simulink model "Proiect_3_sim"  (R2025b)
settings: Solver=VariableStepAuto  StartTime=0.0  StopTime=10.0  RelTol=1e-3
libraries: slpidlib x1
settings Model: Creator=Rares  LastModifiedBy=Rares

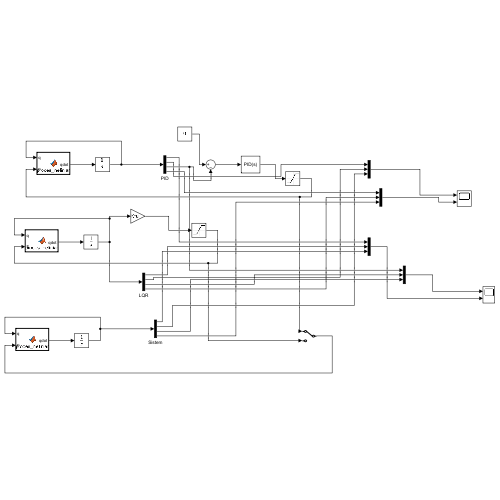
[thumbnail: Simulink's stored preview of the top-level diagram]
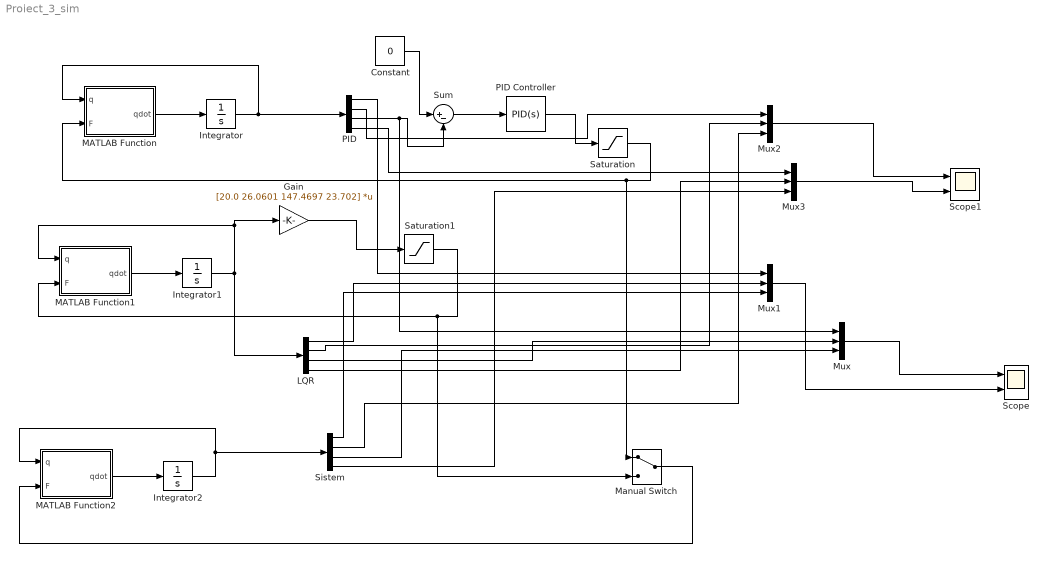
== system Proiect_3_sim ==
  Constant : Constant  Value=0
  Gain : Gain  Gain=[20.0 26.0601 147.4697 23.702]  Multiplication=Matrix(K*u)
  Integrator : Integrator  InitialCondition=[0;0;0.5;0]
  Integrator1 : Integrator  InitialCondition=[0;0;0.5;0]
  Integrator2 : Integrator  InitialCondition=[0;0;0.5;0]
  LQR : Demux
  MATLAB Function : MATLAB Function  TreatAsAtomicUnit=on
  MATLAB Function1 : MATLAB Function  TreatAsAtomicUnit=on
  MATLAB Function2 : MATLAB Function  TreatAsAtomicUnit=on
  Manual Switch : ManualSwitch
  Mux{,1..3} (4 alike) : Mux  Inputs=3
  PID : Demux
  PID Controller : slpidlib/PID Controller  Controller=PID  Form=Parallel  TimeDomain=Continuous-time  UseExternalTs=off  SampleTime=-1  IntegratorMethod=Forward Euler  FilterMethod=Forward Euler  ControllerParametersSource=internal  P=-12.8009  I=-6.9217  UseKiTs=off  D=-1.9402  UseExternalDerivativeSource=off  N=100  UseFilter=on  TunerSelectOption=Transfer Function Based (PID Tuner App)  InitialConditionSource=internal  InitialConditionForIntegrator=0  InitialConditionForFilter=0  DifferentiatorICPrevScaledInput=0  ExternalReset=none  TrackingMode=off  Kt=1  LimitOutput=off  SatLimitsSource=internal  UpperSaturationLimit=inf  LowerSaturationLimit=-inf  LinearizeAsGain=on  AntiWindupMode=none  Kb=1  LimitIntegrator=off  UpperIntegratorSaturationLimit=inf  LowerIntegratorSaturationLimit=-inf  POutMin=[]  POutMax=[]  IOutMin=[]  IOutMax=[]  DOutMin=[]  DOutMax=[]  NOutMin=[]  NOutMax=[]  SumOutMin=[]  SumOutMax=[]  SaturationOutMin=[]  SaturationOutMax=[]  PParamMin=[]  PParamMax=[]  IParamMin=[]  IParamMax=[]  DParamMin=[]  DParamMax=[]  NParamMin=[]  NParamMax=[]  KbParamMin=[]  KbParamMax=[]  KtParamMin=[]  KtParamMax=[]  KbOutMin=[]  KbOutMax=[]  KtOutMin=[]  KtOutMax=[]  IntegratorOutMin=[]  IntegratorOutMax=[]  FilterOutMin=[]  FilterOutMax=[]  SumI1OutMin=[]  SumI1OutMax=[]  SumI2OutMin=[]  SumI2OutMax=[]  SumI3OutMin=[]  SumI3OutMax=[]  SumI4OutMin=[]  SumI4OutMax=[]  SumDOutMin=[]  SumDOutMax=[]  DifferentiatorOutMin=[]  DifferentiatorOutMax=[]  FilterDiffOutCoefMin=[]  FilterDiffOutCoefMax=[]  ReciprocalOutMin=[]  ReciprocalOutMax=[]  SumDenOutMin=[]  SumDenOutMax=[]  SumNumOutMin=[]  SumNumOutMax=[]  DivideOutMin=[]  DivideOutMax=[]  UdiffTsProdOutMin=[]  UdiffTsProdOutMax=[]  NTsProdOutMin=[]  NTsProdOutMax=[]  UintegralTsProdOutMin=[]  UintegralTsProdOutMax=[]  UngainTsProdOutMin=[]  UngainTsProdOutMax=[]  ClampingZeroOutDataTypeStr=Inherit: Inherit via back propagation  ClampingZeroOutMin=[]  ClampingZeroOutMax=[]  FilterDenConstantOutDataTypeStr=Inherit: Inherit via back propagation  FilterDenConstantOutMin=[]  FilterDenConstantOutMax=[]  PCopyOutDataTypeStr=Inherit: Inherit via back propagation  PCopyOutMin=[]  PCopyOutMax=[]  NCopyOutDataTypeStr=Inherit: Inherit via back propagation  NCopyOutMin=[]  NCopyOutMax=[]  IntegratorContinuousStateAttributes=''  IntegratorStateMustResolveToSignalObject=off  IntegratorRTWStateStorageClass=Auto  FilterContinuousStateAttributes=''  FilterStateMustResolveToSignalObject=off  FilterRTWStateStorageClass=Auto  ParallelPVariant=InternalParameters  IdealPVariant=Disabled  IVariant=InternalParameters  DVariant=InternalParameters  IntegratorVariant=Continuous  SatVariant=Disabled  AWVariant=Passthrough  PCopyVariant=Disabled  TRVariant=Disabled  FdbkBlocksVariant=Forward  IdealPFdbkVariant=Disabled  SatFdbkVariant=Disabled  DerivativeFilterVariant=ContFilter  NVariant=InternalParameters  NCopyVariant=Disabled  FilterICVariant=InternalICsFilter  IntegratorICVariant=InternalICs  ExternalResetVariant=Disabled  TRSumVariant=Passthrough  SumFdbkVariant=Disabled  SumVariant=Sum_PID  TsampFilterVariant=InternalTs  TsampNgainVariant=Passthrough  TsampIntegralVariant=Disabled_SignalSpec  ExternalSaturationOutDataTypeStr=Inherit: Same as second input  DerivativeSourceVariant=ErrorSignal  PreIntVariant=InternalPreInt
  Saturation : Saturate  UpperLimit=10  LowerLimit=-10
  Saturation1 : Saturate  UpperLimit=10  LowerLimit=-10
  Scope : Scope  NumInputPorts=2
      settings: ActiveDisplayYMinimum=-0.23429520453930819  ActiveDisplayYMaximum=0.5815883560599231
  Scope1 : Scope  NumInputPorts=2
      settings: ActiveDisplayYMinimum=-4.4566103795185814  ActiveDisplayYMaximum=2.4235967168961703
  Sistem : Demux
  Sum : Sum  Inputs=|+-
  wires:
  MATLAB Function/1(qdot) -> Integrator/1
  Integrator/1 -> PID/1, MATLAB Function/1(q)
  Constant/1 -> Sum/1
  PID/3 -> Mux/1, Sum/2
  PID Controller/1 -> Saturation/1
  Saturation/1 -> Manual Switch/1, MATLAB Function/2(F)
  Sum/1 -> PID Controller/1
  Integrator1/1 -> Gain/1, MATLAB Function1/1(q), LQR/1
  MATLAB Function1/1(qdot) -> Integrator1/1
  Gain/1 -> Saturation1/1
  Saturation1/1 -> Manual Switch/2, MATLAB Function1/2(F)
  MATLAB Function2/1(qdot) -> Integrator2/1
  Integrator2/1 -> Sistem/1, MATLAB Function2/1(q)
  Manual Switch/1 -> MATLAB Function2/2(F)
  LQR/3 -> Mux/2
  Mux/1 -> Scope/1
  PID/1 -> Mux1/1
  LQR/1 -> Mux1/2
  PID/2 -> Mux2/1
  LQR/2 -> Mux2/2
  Sistem/2 -> Mux2/3
  Mux2/1 -> Scope1/1
  PID/4 -> Mux3/1
  LQR/4 -> Mux3/2
  Sistem/4 -> Mux3/3
  Mux3/1 -> Scope1/2
  Mux1/1 -> Scope/2
  Sistem/1 -> Mux1/3
  Sistem/3 -> Mux/3

== matlab function Proiect_3_sim/MATLAB Function ==
  data: q input; qdot output; F input
function qdot = proces_neliniar(q, F)
Mc = 0.5; m = 0.2; l = 0.3; D = 0.1; g = 9.8;
x = q(1); xdot = q(2); theta = q(3); thetadot = q(4);

s = sin(theta); c = cos(theta);
Delta = Mc + m*s^2;
xddot = ( F - D*xdot + m*l*thetadot^2*s - m*g*s*c ) / (Mc + m*s^2);
thetaddot = ( (Mc+m)*g*s - c*(F - D*xdot + m*l*thetadot^2*s) ) / (l*(Mc + m*s^2));

qdot = [xdot; xddot; thetadot; thetaddot];
end

== matlab function Proiect_3_sim/MATLAB Function2 ==
  data: q input; qdot output; F input
function qdot = proces_neliniar(q, F)
Mc = 0.5; m = 0.2; l = 0.3; D = 0.1; g = 9.8;
x = q(1); xdot = q(2); theta = q(3); thetadot = q(4);

s = sin(theta); c = cos(theta);
Delta = Mc + m*s^2;
xddot = ( F - D*xdot + m*l*thetadot^2*s - m*g*s*c ) / (Mc + m*s^2);
thetaddot = ( (Mc+m)*g*s - c*(F - D*xdot + m*l*thetadot^2*s) ) / (l*(Mc + m*s^2));

qdot = [xdot; xddot; thetadot; thetaddot];
end

== matlab function Proiect_3_sim/MATLAB Function1 ==
  data: q input; qdot output; F input
function qdot = proces_neliniar(q, F)
Mc = 0.5; m = 0.2; l = 0.3; D = 0.1; g = 9.8;
x = q(1); xdot = q(2); theta = q(3); thetadot = q(4);

s = sin(theta); c = cos(theta);
Delta = Mc + m*s^2;
xddot = ( F - D*xdot + m*l*thetadot^2*s - m*g*s*c ) / (Mc + m*s^2);
thetaddot = ( (Mc+m)*g*s - c*(F - D*xdot + m*l*thetadot^2*s) ) / (l*(Mc + m*s^2));

qdot = [xdot; xddot; thetadot; thetaddot];
end
